simulink model "MaskDemo"  (R2014a)
settings: Solver=ode3  StartTime=0.0  StopTime=10.0  FixedStep=0.01  RelTol=1e-3
settings Model: Creator=李广文  LastModifiedBy=李广文

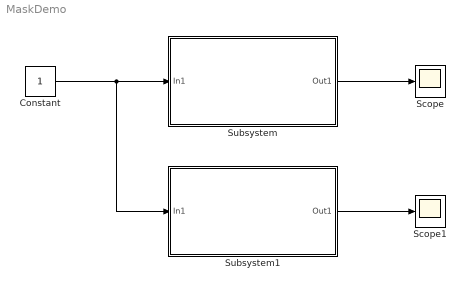
== system MaskDemo ==
  Constant : Constant
  Scope : Scope
  Scope1 : Scope
  Subsystem : Subsystem  mask{Kp=10, Ki=0, Kd=0.5}
      mask prompts: Kp "比例系数"; Ki "积分系数"; Kd "微分系数"
      mask Display: text(-100,-100, '别动我！！！')
  Subsystem1 : Subsystem  mask{Kp1=15.800, Ki1=1.000, Kd1=1.000}
      mask prompts: Kp1 "比例"; Ki1 "积分"; Kd1 "微分"
      mask DialogControl DescTextVar Prompt: 别改
  wires:
  Subsystem/1(Out1) -> Scope/1
  Constant/1 -> Subsystem1/1(In1), Subsystem/1(In1)
  Subsystem1/1(Out1) -> Scope1/1

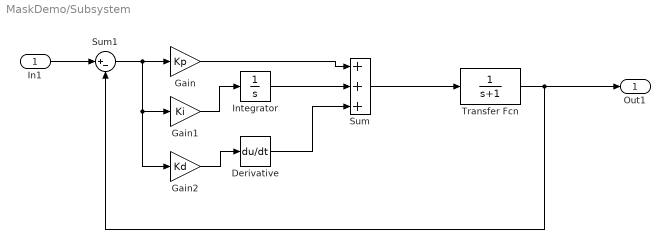
== system MaskDemo/Subsystem ==
  In1 : Inport
  Derivative : Derivative
  Gain : Gain  Gain=Kp
  Gain1 : Gain  Gain=Ki
  Gain2 : Gain  Gain=Kd
  Integrator : Integrator
  Sum : Sum  Inputs=+++
  Sum1 : Sum  Inputs=|+-
  Transfer Fcn : TransferFcn  Denominator=[1 1]
  Out1 : Outport
  wires:
  Gain2/1 -> Derivative/1
  Gain/1 -> Sum/1
  Integrator/1 -> Sum/2
  Derivative/1 -> Sum/3
  Gain1/1 -> Integrator/1
  Sum/1 -> Transfer Fcn/1
  Transfer Fcn/1 -> Sum1/2, Out1/1
  In1/1 -> Sum1/1
  Sum1/1 -> Gain2/1, Gain1/1, Gain/1

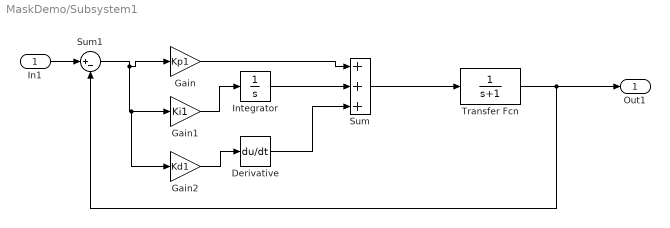
== system MaskDemo/Subsystem1 ==
  In1 : Inport
  Derivative : Derivative
  Gain : Gain  Gain=Kp1
  Gain1 : Gain  Gain=Ki1
  Gain2 : Gain  Gain=Kd1
  Integrator : Integrator
  Sum : Sum  Inputs=+++
  Sum1 : Sum  Inputs=|+-
  Transfer Fcn : TransferFcn  Denominator=[1 1]
  Out1 : Outport
  wires:
  Transfer Fcn/1 -> Sum1/2, Out1/1
  Sum/1 -> Transfer Fcn/1
  Gain1/1 -> Integrator/1
  Derivative/1 -> Sum/3
  Integrator/1 -> Sum/2
  Gain/1 -> Sum/1
  Gain2/1 -> Derivative/1
  Sum1/1 -> Gain2/1, Gain1/1, Gain/1
  In1/1 -> Sum1/1
